simulink library "libCM"  (R2022b)
settings: Solver=VariableStepAuto  StartTime=0.0  StopTime=10.0  RelTol=1e-3
libraries: simulink x6
settings Model: Creator=NurdoganUrbanMobilit  LastModifiedBy=NurdoganUrbanMobilit

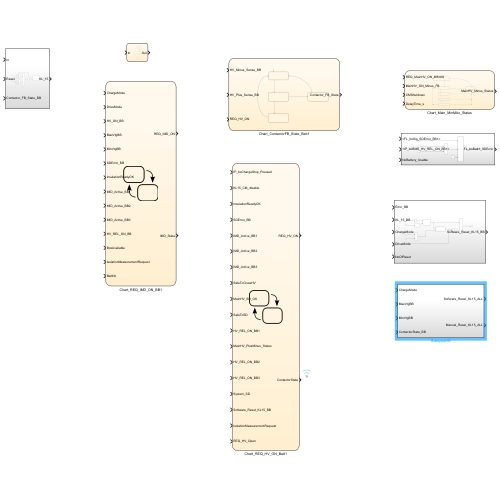
[thumbnail: Simulink's stored preview of the top-level diagram]
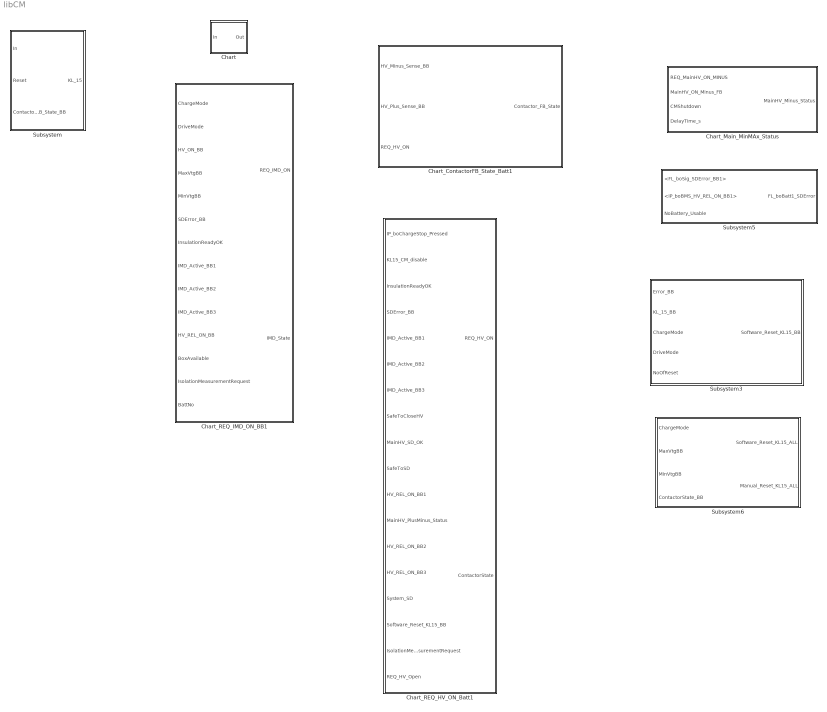
== system libCM ==
  Chart : Stateflow chart  TreatAsAtomicUnit=on
  Chart_ContactorFB_State_Batt1 : Stateflow chart  TreatAsAtomicUnit=on
      settings: RTWSystemCode=Reusable function  RTWFcnNameOpts=Use subsystem name  RTWFileNameOpts=Use subsystem name
  Chart_Main_MinMAx_Status : Stateflow chart
      settings: RTWSystemCode=Reusable function  RTWFcnNameOpts=Use subsystem name  RTWFileNameOpts=Use subsystem name  PortSchema="{\"entries\":[{\"content\":{\"sides\":[{\"content\":{\"connectorIds\":[\"In1\",\"In2\",\"In4\",\"In3\"]},\"type\":\"ConnectorPlacement.EquallySpacedRectSide\",\"uuid\":\"af513ad7-882d-44ca-bd16-f13375ad0cc7\"},{\"content\":{\"connectorIds\":[\"Out1\"],\"side\":\"RIGHT\"},\"type\":\"ConnectorPlacement.EquallySpacedRectSide\",\"uuid\":\"1e07241b-ff1c-4b1c-99ea-8f556d1f4bde\"},{\"content\":{\"connectorIds\":[],\"side\":\"TOP\"},\"type\":\"ConnectorPlacement.EquallySpacedRectSide\",\"uuid\":\"c2fbf455-7245-4f9b-917b-4eed34a267cf\"}]},\"type\":\"ConnectorPlacement.EquallySpacedConnector\",\"uuid\":\"56193be1-d801-449e-8417-1819ff958dca\"}],\"packageUris\":[\"http://schema.mathworks.com/mf0/Connector/R2020b\"],\"version\":\"1.0\"}"
  Chart_REQ_HV_ON_Batt1 : Stateflow chart  TreatAsAtomicUnit=on
      settings: RTWSystemCode=Reusable function  RTWFcnNameOpts=Use subsystem name  RTWFileNameOpts=Use subsystem name  PortSchema="{\"entries\":[{\"content\":{\"sides\":[{\"content\":{\"connectorIds\":[\"In1\",\"In8\",\"In2\",\"In3\",\"In4\",\"In5\",\"In6\",\"In9\",\"In10\",\"In11\",\"In15\",\"In16\",\"In12\",\"In13\",\"In14\",\"In7\",\"In17\",\"In18\"]},\"type\":\"ConnectorPlacement.EquallySpacedRectSide\",\"uuid\":\"2be98496-94d0-443a-935f-4b2e992aab8e\"},{\"content\":{\"connectorIds\":[\"Out1\",\"Out2\"],\"side\":\"RIGHT\"},\"type\":\"ConnectorPlacement.EquallySpacedRectSide\",\"uuid\":\"fda23760-2911-4bbb-ac8a-7a2dd70a4d72\"},{\"content\":{\"connectorIds\":[],\"side\":\"TOP\"},\"type\":\"ConnectorPlacement.EquallySpacedRectSide\",\"uuid\":\"77874347-bb9f-447e-8cfd-08f52997a658\"}]},\"type\":\"ConnectorPlacement.EquallySpacedConnector\",\"uuid\":\"fcafe625-79d7-4037-9431-d1cc167f79ab\"}],\"packageUris\":[\"http://schema.mathworks.com/mf0/Connector/R2020b\"],\"version\":\"1.0\"}"
  Chart_REQ_IMD_ON_BB1 : Stateflow chart  TreatAsAtomicUnit=on
      settings: RTWSystemCode=Reusable function  RTWFcnNameOpts=Use subsystem name  RTWFileNameOpts=Use subsystem name  PortSchema="{\"entries\":[{\"content\":{\"sides\":[{\"content\":{\"connectorIds\":[\"In1\",\"In2\",\"In8\",\"In4\",\"In5\",\"In6\",\"In3\",\"In11\",\"In9\",\"In10\",\"In12\",\"In13\",\"In14\",\"In7\"]},\"type\":\"ConnectorPlacement.EquallySpacedRectSide\",\"uuid\":\"8d42b6d3-700d-4664-9176-2af1fd91a5ef\"},{\"content\":{\"connectorIds\":[\"Out1\",\"Out2\"],\"side\":\"RIGHT\"},\"type\":\"ConnectorPlacement.EquallySpacedRectSide\",\"uuid\":\"1055ad88-7b4e-4849-9034-0e2b968d970a\"},{\"content\":{\"connectorIds\":[],\"side\":\"TOP\"},\"type\":\"ConnectorPlacement.EquallySpacedRectSide\",\"uuid\":\"93b8508a-130b-4038-9854-7181d979ecdb\"}]},\"type\":\"ConnectorPlacement.EquallySpacedConnector\",\"uuid\":\"712ba1bb-a03e-4078-b3d0-f15207ecb0ed\"}],\"packageUris\":[\"http://schema.mathworks.com/mf0/Connector/R2020b\"],\"version\":\"1.0\"}"
  Subsystem : Subsystem
  Subsystem3 : Subsystem
  Subsystem5 : Subsystem
  Subsystem6 : Subsystem

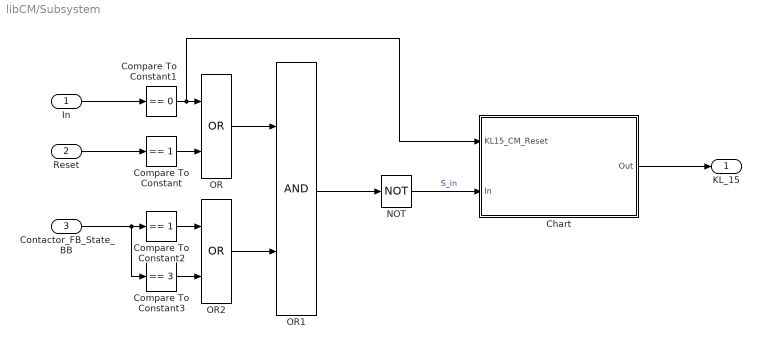
== system libCM/Subsystem ==
  In : Inport
  Reset : Inport  Port=2
  Contactor_FB_State_BB : Inport  Port=3
  Chart : Stateflow chart
      settings: PortSchema="{\"entries\":[{\"content\":{\"sides\":[{\"content\":{\"connectorIds\":[\"In2\",\"In1\"]},\"type\":\"ConnectorPlacement.EquallySpacedRectSide\",\"uuid\":\"43c02b2f-207c-4b5f-80bd-d1d7ba59fb15\"},{\"content\":{\"connectorIds\":[\"Out1\"],\"side\":\"RIGHT\"},\"type\":\"ConnectorPlacement.EquallySpacedRectSide\",\"uuid\":\"d486706b-7d54-4899-a5ac-d6954abb568f\"},{\"content\":{\"connectorIds\":[],\"side\":\"TOP\"},\"type\":\"ConnectorPlacement.EquallySpacedRectSide\",\"uuid\":\"195c5d35-20b5-45e8-8e51-8d3e77e84cc9\"}]},\"type\":\"ConnectorPlacement.EquallySpacedConnector\",\"uuid\":\"336c13ab-07c5-4b2d-9c13-20514a94ff2c\"}],\"packageUris\":[\"http://schema.mathworks.com/mf0/Connector/R2020b\"],\"version\":\"1.0\"}"
  Compare To Constant : simulink/Logic and Bit Operations/Compare To Constant  relop===  const=1  OutDataTypeStr=boolean
  Compare To Constant1 : simulink/Logic and Bit Operations/Compare To Constant  relop===  const=0  OutDataTypeStr=boolean
  Compare To Constant2 : simulink/Logic and Bit Operations/Compare To Constant  relop===  const=1  OutDataTypeStr=boolean
  Compare To Constant3 : simulink/Logic and Bit Operations/Compare To Constant  relop===  const=3  OutDataTypeStr=boolean
  NOT : Logic  Operator=NOT  AllPortsSameDT=off  OutDataTypeStr=boolean
  OR : Logic  Operator=OR  AllPortsSameDT=off  OutDataTypeStr=boolean
  OR1 : Logic  AllPortsSameDT=off  OutDataTypeStr=boolean
  OR2 : Logic  Operator=OR  AllPortsSameDT=off  OutDataTypeStr=boolean
  KL_15 : Outport
  wires:
  Compare To Constant1/1 -> Chart/2(KL15_CM_Reset), OR/1
  Reset/1 -> Compare To Constant/1
  Compare To Constant3/1 -> OR2/2
  Compare To Constant2/1 -> OR2/1
  Contactor_FB_State_BB/1 -> Compare To Constant3/1, Compare To Constant2/1
  In/1 -> Compare To Constant1/1
  Compare To Constant/1 -> OR/2
  OR1/1 -> NOT/1
  Chart/1(Out) -> KL_15/1
  OR/1 -> OR1/1
  OR2/1 -> OR1/2
  NOT/1 -> Chart/1(In)  "S_in"

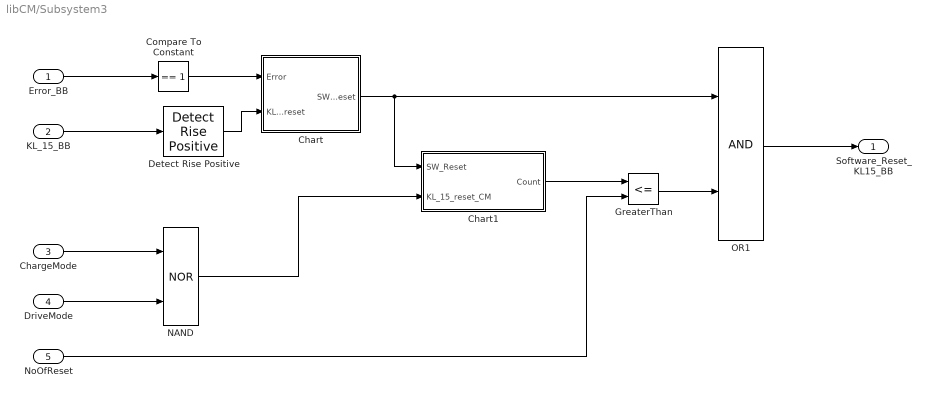
== system libCM/Subsystem3 ==
  Error_BB : Inport
  KL_15_BB : Inport  Port=2
  ChargeMode : Inport  Port=3
  DriveMode : Inport  Port=4
  NoOfReset : Inport  Port=5
  Chart : Stateflow chart
  Chart1 : Stateflow chart
  Compare To Constant : simulink/Logic and Bit Operations/Compare To Constant  relop===  const=1  OutDataTypeStr=boolean
  Detect Rise Positive : simulink/Logic and Bit Operations/Detect Rise Positive  vinit=0  OutDataTypeStr=boolean
  GreaterThan : RelationalOperator  Operator=<=  OutDataTypeStr=boolean  RndMeth=Simplest  InputSameDT=off
  NAND : Logic  Operator=NOR  AllPortsSameDT=off  OutDataTypeStr=boolean
  OR1 : Logic  AllPortsSameDT=off  OutDataTypeStr=boolean
  Software_Reset_KL15_BB : Outport
  wires:
  DriveMode/1 -> NAND/2
  GreaterThan/1 -> OR1/2
  Detect Rise Positive/1 -> Chart/2(KL15_reset)
  ChargeMode/1 -> NAND/1
  Compare To Constant/1 -> Chart/1(Error)
  OR1/1 -> Software_Reset_KL15_BB/1
  Error_BB/1 -> Compare To Constant/1
  NoOfReset/1 -> GreaterThan/2
  Chart1/1(Count) -> GreaterThan/1
  Chart/1(SW_Reset) -> Chart1/1(SW_Reset), OR1/1
  KL_15_BB/1 -> Detect Rise Positive/1
  NAND/1 -> Chart1/2(KL_15_reset_CM)

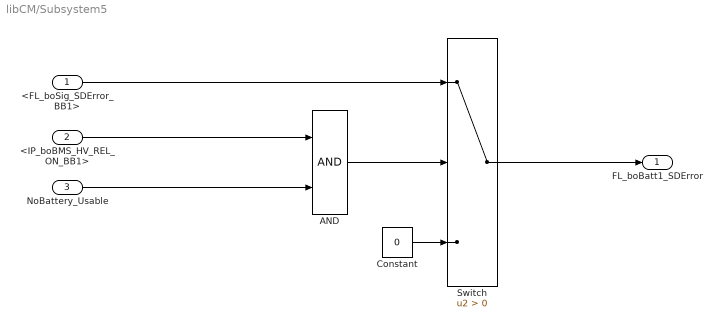
== system libCM/Subsystem5 ==
  <FL_boSig_SDError_BB1> : Inport
  <IP_boBMS_HV_REL_ON_BB1> : Inport  Port=2
  NoBattery_Usable : Inport  Port=3
  AND : Logic  AllPortsSameDT=off  OutDataTypeStr=boolean
  Constant : Constant  Value=0  OutDataTypeStr=boolean
  Switch : Switch  Criteria=u2 > Threshold  SaturateOnIntegerOverflow=off  InputSameDT=off
  FL_boBatt1_SDError : Outport
  wires:
  <FL_boSig_SDError_BB1>/1 -> Switch/1
  Constant/1 -> Switch/3
  NoBattery_Usable/1 -> AND/2
  Switch/1 -> FL_boBatt1_SDError/1
  AND/1 -> Switch/2
  <IP_boBMS_HV_REL_ON_BB1>/1 -> AND/1

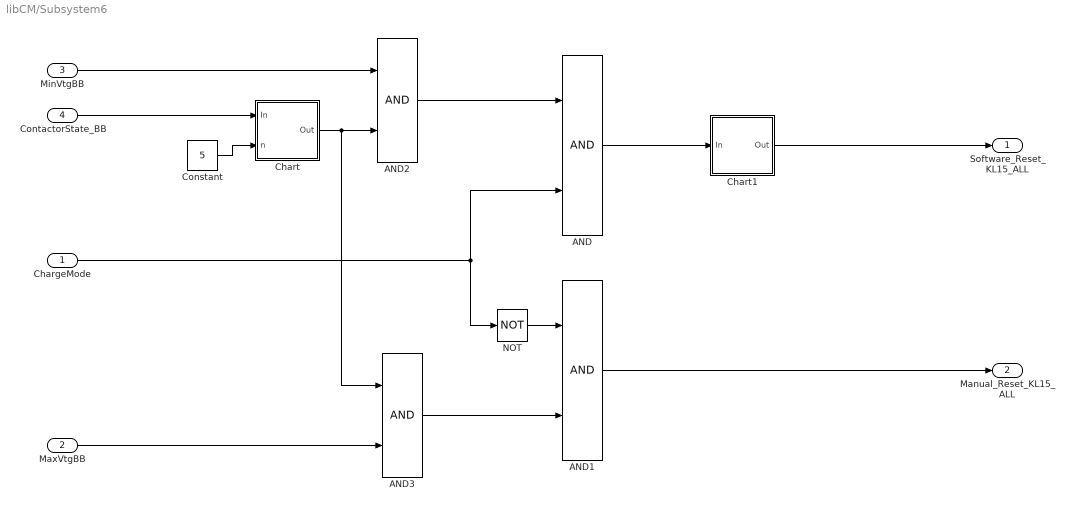
== system libCM/Subsystem6 ==
  ChargeMode : Inport
  MaxVtgBB : Inport  Port=2
  MinVtgBB : Inport  Port=3
  ContactorState_BB : Inport  Port=4
  AND{,1..3} (4 alike) : Logic  AllPortsSameDT=off  OutDataTypeStr=boolean
  Chart : Stateflow chart
  Chart1 : Stateflow chart
  Constant : Constant  Value=5
  NOT : Logic  Operator=NOT  AllPortsSameDT=off  OutDataTypeStr=boolean
  Software_Reset_KL15_ALL : Outport
  Manual_Reset_KL15_ALL : Outport  Port=2
  wires:
  ContactorState_BB/1 -> Chart/1(In)
  AND2/1 -> AND/1
  MinVtgBB/1 -> AND2/1
  ChargeMode/1 -> AND/2, NOT/1
  AND3/1 -> AND1/2
  Chart/1(Out) -> AND3/1, AND2/2
  AND1/1 -> Manual_Reset_KL15_ALL/1
  NOT/1 -> AND1/1
  Constant/1 -> Chart/2(n)
  MaxVtgBB/1 -> AND3/2
  AND/1 -> Chart1/1(In)
  Chart1/1(Out) -> Software_Reset_KL15_ALL/1

== stateflow chart libCM/Chart_REQ_HV_ON_Batt1 ==
  state Default
    REQ_HV_ON = 0
    ContactorState = 1
  state hold
  state CONTACTOR_OFF
    REQ_HV_ON = 0
    ContactorState = 2
  state CONTACTOR_ON
    REQ_HV_ON = 1
    ContactorState = 3
  (default) -> Default
  Default -> CONTACTOR_OFF : [IP_boChargeStop_Pressed == false &&...
      | KL15_CM_disable == false &&...
      | InsulationReadyOK == true &&...
      | SDError_BB == false &&...
      | System_SD == false]
  CONTACTOR_OFF -> Default [order 1] : [InsulationReadyOK == false ||...
      | SDError_BB == true ||...
      | Software_Reset_KL15_BB == true ||...
      | KL15_CM_disable == true]
  CONTACTOR_ON -> Default [order 2] : [SDError_BB == true &&...
      | (HV_REL_ON_BB2 == true || HV_REL_ON_BB3 == true) &&...
      | (SafeToSD == true || HV_REL_ON_BB1 == false)]
  CONTACTOR_ON -> Default [order 3] : [(HV_REL_ON_BB2 == true || HV_REL_ON_BB3 == true) &&...
      | REQ_HV_Open == true]
  hold -> Default : [after(2,sec)]
  CONTACTOR_ON -> hold [order 1] : [(KL15_CM_disable == true || System_SD == true || SDError_BB == true) &&...
      | (MainHV_SD_OK == true || HV_REL_ON_BB1 == false)]
  CONTACTOR_OFF -> CONTACTOR_ON [order 2] : [after(2,sec) &&...
      | IMD_Active_BB1 == true &&...
      | IMD_Active_BB2 == false &&...
      | IMD_Active_BB3 == false &&...
      | MainHV_PlusMinus_Status == 0]
  CONTACTOR_OFF -> CONTACTOR_ON [order 3] : [after(2,sec) &&...
      | IMD_Active_BB1 == false &&...
      | MainHV_PlusMinus_Status == 1 &&...
      | (IMD_Active_BB2 == true || IMD_Active_BB3 ==true || IsolationMeasurementRequest == false) &&...
      | SafeToCloseHV == true]
  data: IP_boChargeStop_Pressed input; InsulationReadyOK input; SDError_BB input; REQ_HV_ON output; IMD_Active_BB1 input; IMD_Active_BB2 input; IMD_Active_BB3 input; ContactorState output; Software_Reset_KL15_BB input; KL15_CM_disable input; SafeToCloseHV input; MainHV_SD_OK input; SafeToSD input; HV_REL_ON_BB2 input; HV_REL_ON_BB3 input; System_SD input; HV_REL_ON_BB1 input; MainHV_PlusMinus_Status input; IsolationMeasurementRequest input; REQ_HV_Open input

== stateflow chart libCM/Chart ==
  state Default
    Out = false
  state Hold
    Out = false
  state Actual
    Out = In
  (default) -> Default
  Actual -> Default : [In==false]
  Hold -> Default [order 2] : [In==false]
  Default -> Hold : [In == true]
  Hold -> Actual [order 1] : after(1,sec)
  data: In input boolean; Out output boolean

== stateflow chart libCM/Chart_REQ_IMD_ON_BB1 ==
  state Default
    REQ_IMD_ON = false;
    IMD_State = uint8(0);
  state CHARGE
    state CHARGE
      REQ_IMD_ON = true;
      IMD_State = uint8(4);
    state IMD_ON
      REQ_IMD_ON = true;
      IMD_State = uint8(5);
    state IMD_OFF
      REQ_IMD_ON = false;
      IMD_State = uint8(6);
    (default) -> CHARGE.CHARGE
    CHARGE.CHARGE -> CHARGE.IMD_OFF [order 2] : [(InsulationReadyOK == true && MinVtgBB ~=  BattNo) ||...
        |  HV_ON_BB == true]
    CHARGE.CHARGE -> CHARGE.IMD_ON [order 1] : [InsulationReadyOK == true &&...
        | MinVtgBB == BattNo &&...
        | HV_ON_BB == false]
    CHARGE.IMD_OFF -> CHARGE.IMD_ON : [MinVtgBB == BattNo &&...
        | IMD_Active_BB1 == false &&...
        | IMD_Active_BB2 == false &&...
        | IMD_Active_BB3 == false &&...
        | IsolationMeasurementRequest == true]
    CHARGE.IMD_ON -> CHARGE.IMD_OFF : [HV_ON_BB == true &&...
        | IsolationMeasurementRequest == false]
  state DRIVE
    state DRIVE
      REQ_IMD_ON = true;
      IMD_State = uint8(1);
    state IMD_ON
      REQ_IMD_ON = true;
      IMD_State = uint8(2);
    state IMD_OFF
      REQ_IMD_ON = false;
      IMD_State = uint8(3);
    (default) -> DRIVE.DRIVE
    DRIVE.DRIVE -> DRIVE.IMD_ON [order 1] : [InsulationReadyOK == true &&...
        | MaxVtgBB == BattNo &&...
        | HV_ON_BB == false]
    DRIVE.DRIVE -> DRIVE.IMD_OFF [order 2] : [(InsulationReadyOK == true && MaxVtgBB ~=  BattNo)  ||...
        | HV_ON_BB == true]
    DRIVE.IMD_OFF -> DRIVE.IMD_ON : [MaxVtgBB == BattNo &&...
        | IMD_Active_BB1 == false &&...
        | IMD_Active_BB2 == false &&...
        | IMD_Active_BB3 == false &&...
        | IsolationMeasurementRequest == true]
    DRIVE.IMD_ON -> DRIVE.IMD_OFF : [HV_ON_BB == true &&...
        | IsolationMeasurementRequest == false]
  (default) -> Default
  Default -> CHARGE [order 1] : [ChargeMode == true && DriveMode == false &&...
      |  SDError_BB == false && BoxAvailable==true]
  CHARGE -> Default : [((ChargeMode == false || DriveMode == true ||...
      |  SDError_BB == true || BoxAvailable==false) &&...
      | HV_REL_ON_BB == false)]
  Default -> DRIVE [order 2] : [DriveMode == true && ChargeMode == false &&...
      |  SDError_BB == false && BoxAvailable==true]
  DRIVE -> Default : [((DriveMode == false || ChargeMode == true ||...
      | SDError_BB == true || BoxAvailable==false) &&...
      | HV_REL_ON_BB == false)]
  data: ChargeMode input; DriveMode input; InsulationReadyOK input; MaxVtgBB input; MinVtgBB input; REQ_IMD_ON output boolean; SDError_BB input; BattNo input; HV_ON_BB input; IMD_Active_BB2 input; IMD_Active_BB3 input; IMD_Active_BB1 input; HV_REL_ON_BB input; BoxAvailable input; IsolationMeasurementRequest input; IMD_State output

== stateflow chart libCM/Subsystem6/Chart ==
  state Default
    Out = false
  state Delay
    Out = false
  state Delay1
    Out = true
  (default) -> Default
  Delay1 -> Default : [In == 3]
  Default -> Delay : [In == 2]
  Delay -> Default [order 2] : [In == 1 ||...
      | In == 3]
  Delay -> Delay1 [order 1] : after(n,sec)
  data: In input; Out output; n input

== stateflow chart libCM/Subsystem3/Chart ==
  state Default
    SW_Reset = false
  state KL15_reset
    SW_Reset = false
  state pulse
    SW_Reset = false
  state hold
    SW_Reset = false
  state Delay
    SW_Reset = true
  (default) -> Default
  KL15_reset -> Default : [after(25,sec) &&...
      | Error == false]
  Default -> hold : [Error == true]
  hold -> Default [order 2] : [Error == false]
  pulse -> KL15_reset : [KL15_reset == true]
  Delay -> pulse : [after(10,msec)]
  hold -> Delay [order 1] : after(5,sec)
  data: Error input; SW_Reset output; KL15_reset input

== stateflow chart libCM/Subsystem3/Chart1 ==
  state Default
    Count = 0
  state Delay1
  state Delay
    Count = Count + 1
  (default) -> Default
  Default -> Delay : [SW_Reset == true]
  Delay1 -> Default [order 1] : [KL_15_reset_CM == true]
  Delay1 -> Delay [order 2] : [SW_Reset == true]
  Delay -> Delay1 : [SW_Reset == false]
  data: SW_Reset input; KL_15_reset_CM input; Count output

== stateflow chart libCM/Subsystem6/Chart1 ==
  state Default
    Out = false
  state Delay
    Out = true
  state pulse
    Out = false
  (default) -> Default
  Default -> Delay : [In == true]
  Delay -> pulse : [after(10,msec)]
  data: In input; Out output

== stateflow chart libCM/Chart_ContactorFB_State_Batt1 ==
  state default
    Contactor_FB_State = 0
  state hold
    Contactor_FB_State = 0
  state Error
    Contactor_FB_State = 3
  state Open
    Contactor_FB_State = 1
  (default) -> default
  Open -> default : [REQ_HV_ON == 1]
  Error -> default : [REQ_HV_ON == 1]
  default -> hold : [REQ_HV_ON == 0]
  hold -> Error [order 1] : after(5,sec)
  hold -> Open [order 2] : [HV_Plus_Sense_BB == false &&...
      | HV_Minus_Sense_BB == false]
  data: Contactor_FB_State output; HV_Minus_Sense_BB input; HV_Plus_Sense_BB input; REQ_HV_ON input

== stateflow chart libCM/Chart_Main_MinMAx_Status ==
  state Default
    MainHV_Minus_Status = 0
  state Error
    MainHV_Minus_Status = 3
  state hold
    MainHV_Minus_Status = 0
  state open
    MainHV_Minus_Status = 1
  state hold1
    MainHV_Minus_Status = 1
  state closed
    MainHV_Minus_Status = 2
  (default) -> Default
  Error -> Default : [CMShutdown == true]
  Default -> hold : [REQ_MainHV_ON_MINUS == false &&...
      | CMShutdown == false]
  (junction 48) -> hold
  hold -> Error [order 2] : after(DelayTime_s,sec)
  (junction 43) -> (junction 48)
  hold -> open [order 1] : [MainHV_ON_Minus_FB == false]
  (junction 28) -> Error
  open -> (junction 28) [order 2] : [MainHV_ON_Minus_FB == true]
  (junction 25) -> (junction 28)
  open -> hold1 [order 1] : [REQ_MainHV_ON_MINUS == true]
  hold1 -> (junction 25) [order 2] : after(DelayTime_s,sec)
  (junction 40) -> (junction 25)
  hold1 -> closed [order 1] : [MainHV_ON_Minus_FB == true]
  closed -> (junction 43) [order 1] : [REQ_MainHV_ON_MINUS == false]
  closed -> (junction 40) [order 2] : [MainHV_ON_Minus_FB == false]
  data: REQ_MainHV_ON_MINUS input; MainHV_ON_Minus_FB input; MainHV_Minus_Status output; DelayTime_s input; CMShutdown input boolean

== stateflow chart libCM/Subsystem/Chart ==
  state Default
    Out = false
  state hold
    Out = In
  (default) -> Default
  Default -> hold : [KL15_CM_Reset == false &&...
      | after(100,msec)]
  data: In input; Out output; KL15_CM_Reset input
